simulink model "zad3_3_1_d"  (Simulink 6.5)
settings: Solver=ode45  StartTime=0.0  StopTime=10.0  RelTol=1e-3
settings Model: Creator=rr44283  LastModifiedBy=rr44283

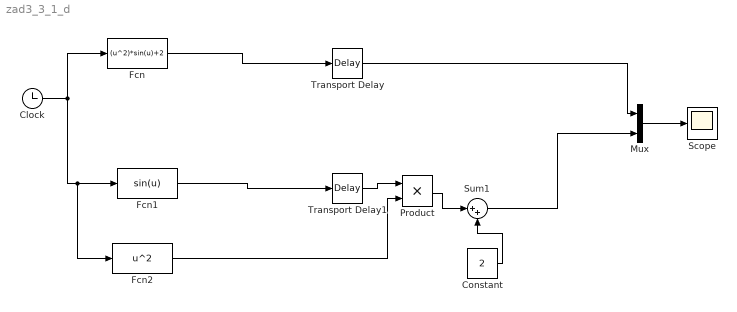
== system zad3_3_1_d ==
  Clock : Clock
      settings: Decimation=10
  Constant : Constant  Value=2  OutDataType=sfix(16)  ConRadixGroup=Use specified scaling  OutScaling=2^0  SampleTime=inf  FramePeriod=inf
  Fcn : Fcn  Expr=(u^2)*sin(u)+2
  Fcn1 : Fcn  Expr=sin(u)
  Fcn2 : Fcn  Expr=u^2
  Mux : Mux  Inputs=2
  Product : Product  RndMeth=Zero
  Scope : Scope
  Sum1 : Sum  Inputs=|++
  Transport Delay : TransportDelay
  Transport Delay1 : TransportDelay
  wires:
  Clock/1 -> Fcn/1, Fcn1/1, Fcn2/1
  Mux/1 -> Scope/1
  Fcn/1 -> Transport Delay/1
  Transport Delay/1 -> Mux/1
  Fcn1/1 -> Transport Delay1/1
  Transport Delay1/1 -> Product/1
  Fcn2/1 -> Product/2
  Product/1 -> Sum1/1
  Constant/1 -> Sum1/2
  Sum1/1 -> Mux/2
